simulink model "model10"  (R2022b)
settings: Solver=ode45  StartTime=0.0  StopTime=10000.0  RelTol=1e-3  EnableMultiTasking=on
libraries: simulink x1
settings Model: Creator=user  LastModifiedBy=lizey
settings SolverCC: AlgebraicLoopSolver=TrustRegion
settings DataIOCC: LimitDataPoints=on  SaveFormat=Array  ReturnWorkspaceOutputs=off
settings OptimizationCC: LifeSpan=inf
settings DebuggingCC: UnconnectedInputMsg=warning  UnconnectedOutputMsg=warning  UnconnectedLineMsg=warning  SFUnexpectedBacktrackingDiag=warning  SFNoUnconditionalDefaultTransitionDiag=warning  SFExecutionAtInitializationDiag=none  SFMachineParentedDataDiag=warning  ArithmeticOperatorsInVariantConditions=warning
settings HardwareCC: ProdBitPerPointer=32  ProdBitPerSizeT=32  ProdBitPerPtrDiffT=32  ProdLargestAtomicFloat=None  ProdIntDivRoundTo=Undefined  ProdEndianess=Unspecified  ProdWordSize=32  ProdHWDeviceType=32-bit Generic
settings ModelReferenceCC: PropagateSignalLabelsOutOfModel=off
settings SFSimCC: SimUseLocalCustomCode=off  CustomCodeUndefinedFunction=UseInterfaceOnly
settings RTWCC: RTWUseLocalCustomCode=off
settings CodeAppCC: StateflowObjectComments=on
settings GRTTargetCC: TargetLangStandard=C89/C90 (ANSI)
settings ConfigComp: CovMetricSettings=dw  CovSaveCumulativeToWorkspaceVar=on  CovSaveSingleToWorkspaceVar=on  CovExternalEMLEnable=off

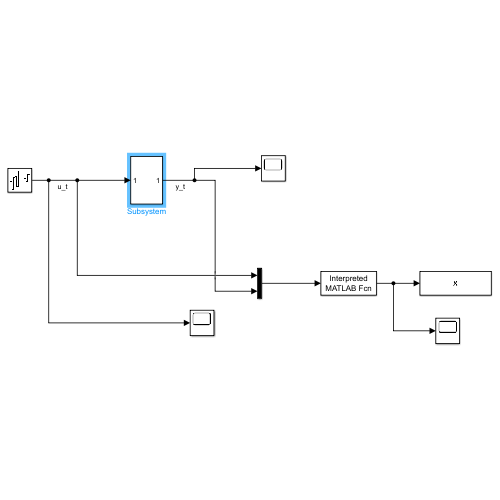
[thumbnail: Simulink's stored preview of the top-level diagram]
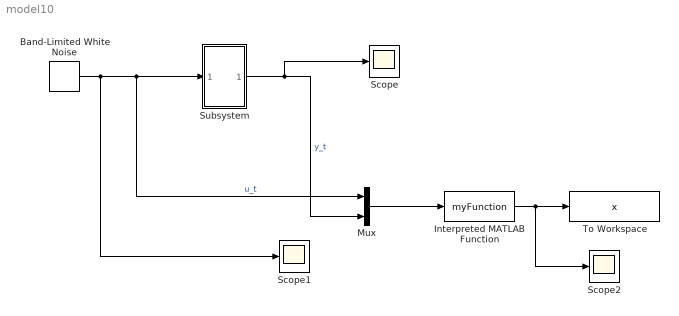
== system model10 ==
  Band-Limited White Noise : simulink/Sources/Band-Limited White Noise  Cov=[0.1]  Ts=1  seed=[23341]
  Interpreted MATLAB Function : MATLABFcn  MATLABFcn=myFunction
  Mux : Mux  Inputs=2
  Scope : Scope
  Scope1 : Scope
  Scope2 : Scope
  Subsystem : Subsystem
  To Workspace : ToWorkspace  VariableName=x  SaveFormat=Timeseries  SampleTime=1
  wires:
  Band-Limited White Noise/1 -> Scope1/1, Mux/1, Subsystem/1(In1)  "u_t"
  Subsystem/1(Out1) -> Scope/1, Mux/2  "y_t"
  Mux/1 -> Interpreted MATLAB Function/1
  Interpreted MATLAB Function/1 -> Scope2/1, To Workspace/1

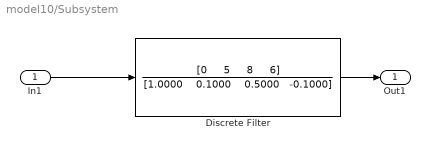
== system model10/Subsystem ==
  In1 : Inport
  Discrete Filter : DiscreteFilter  Numerator="[0     5     8     6]"  Denominator="[1.0000    0.1000    0.5000   -0.1000]"  SampleTime=1
  Out1 : Outport
  wires:
  In1/1 -> Discrete Filter/1
  Discrete Filter/1 -> Out1/1
